simulink model "NewModel"  (R2018a)
settings: Solver=VariableStepAuto  StartTime=0.0  StopTime=10  RelTol=1e-3
values from neighbouring files (symbols this model uses):
  a22 = -2*beta*(c+f10)/numitor    (= -0.0723201373103)    [Proiect_script_IRA2.m]    (also in decupalre.m; trying.m)
  a23 = -M*g*L*f10/numitor    (= -43.7694067093)    [Proiect_script_IRA2.m]    (also in decupalre.m; trying.m)
  a24 = 2*beta*(c+f10)/numitor    (= 0.0723201373103)    [Proiect_script_IRA2.m]    (also in decupalre.m; trying.m)
  a42 = 2*beta*(d+f10)/numitor    (= 0.0279773616358)    [Proiect_script_IRA2.m]    (also in decupalre.m; trying.m)
  a43 = d*M*g*L/numitor    (= 43.7747367103)    [Proiect_script_IRA2.m]    (also in decupalre.m; trying.m)
  a44 = 2*beta*(d+f10)/numitor    (= 0.0279773616358)    [Proiect_script_IRA2.m]    (also in decupalre.m = -0.0279773616358; trying.m = -0.0279773616358)
  a66 = ((-W*W*beta)/(2*R*R))/(m*W*W/2+W*W/(2*R*R)*(Jw+Jm)+Jphi)    (= -0.112438053457)    [Proiect_script_IRA2.m]    (also in decupalre.m; trying.m)
  b21 = alfa*(c+f10)/numitor    (= 1.04508868945)    [Proiect_script_IRA2.m]    (also in decupalre.m; trying.m)
  b22 = alfa*(c+f10)/numitor    (= 1.04508868945)    [Proiect_script_IRA2.m]    (also in decupalre.m; trying.m)
  b41 = -alfa*(d+f10)/numitor    (= -0.404297133465)    [Proiect_script_IRA2.m]    (also in decupalre.m; trying.m)
  b42 = -alfa*(d+f10)/numitor    (= -0.404297133465)    [Proiect_script_IRA2.m]    (also in decupalre.m; trying.m)
  b61 = ((-W*alfa)/(2*R))/(m*W*W/2+W*W/(2*R*R)*(Jw+Jm)+Jphi)    (= -0.609310260785)    [Proiect_script_IRA2.m]    (also in decupalre.m; trying.m)
  b62 = ((-W*alfa)/(2*R))/(m*W*W/2+W*W/(2*R*R)*(Jw+Jm)+Jphi)    (= -0.609310260785)    [Proiect_script_IRA2.m]    (also in decupalre.m; trying.m)
settings Model: Creator=Andrei  LastModifiedBy=Andrei

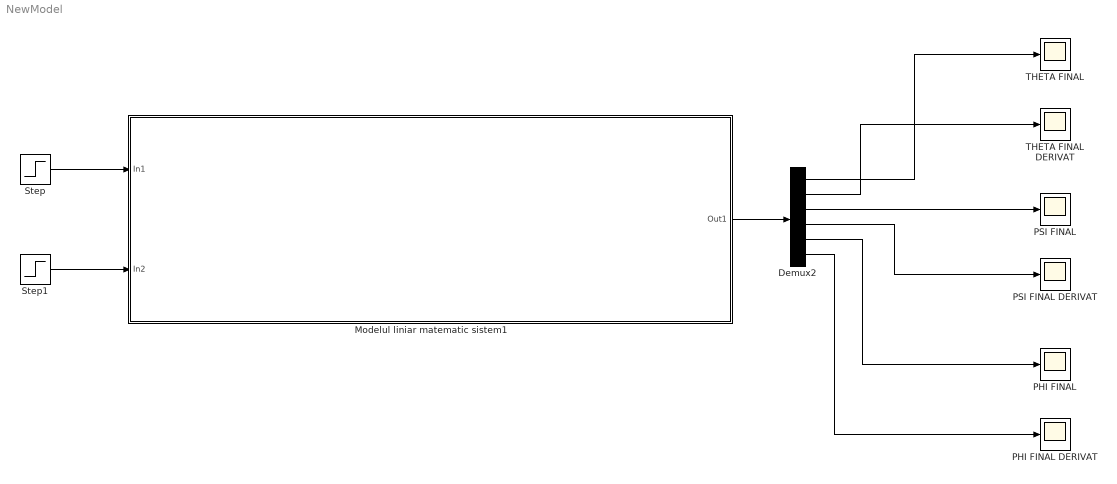
== system NewModel ==
  Demux2 : Demux  Outputs=6
  Modelul liniar matematic sistem1 : Subsystem
  PHI FINAL : Scope
  "PHI FINAL DERIVAT " : Scope
  PSI FINAL : Scope
  "PSI FINAL DERIVAT " : Scope
  Step : Step  Time=0  SampleTime=0
  Step1 : Step  Time=0  SampleTime=0
  THETA FINAL : Scope
  "THETA FINAL DERIVAT " : Scope
  wires:
  Demux2/1 -> THETA FINAL/1
  Demux2/2 -> "THETA FINAL DERIVAT "/1
  Demux2/3 -> PSI FINAL/1
  Modelul liniar matematic sistem1/1(Out1) -> Demux2/1
  Demux2/4 -> "PSI FINAL DERIVAT "/1
  Demux2/6 -> "PHI FINAL DERIVAT "/1
  Demux2/5 -> PHI FINAL/1
  Step/1 -> Modelul liniar matematic sistem1/1(In1)
  Step1/1 -> Modelul liniar matematic sistem1/2(In2)

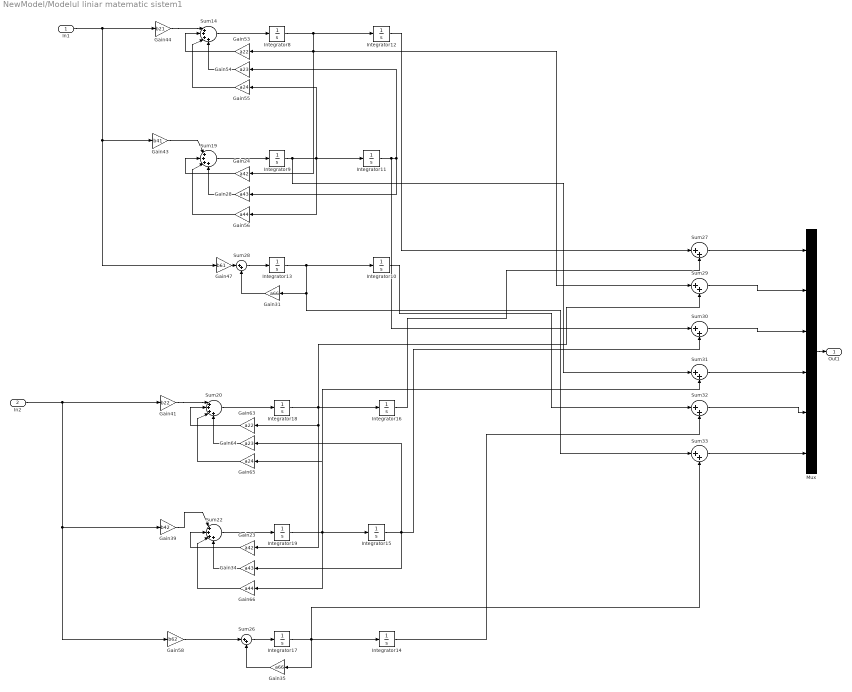
== system NewModel/Modelul liniar matematic sistem1 ==
  In1 : Inport
  In2 : Inport  Port=2
  Gain23 : Gain  Gain=a42
  Gain24 : Gain  Gain=a42
  Gain28 : Gain  Gain=a43
  Gain31 : Gain  Gain=a66
  Gain34 : Gain  Gain=a43
  Gain35 : Gain  Gain=a66
  Gain39 : Gain  Gain=b42
  Gain41 : Gain  Gain=b22
  Gain43 : Gain  Gain=b41
  Gain44 : Gain  Gain=b21
  Gain47 : Gain  Gain=b61
  Gain53 : Gain  Gain=a22
  Gain54 : Gain  Gain=a23
  Gain55 : Gain  Gain=a24
  Gain56 : Gain  Gain=a44
  Gain58 : Gain  Gain=b62
  Gain63 : Gain  Gain=a22
  Gain64 : Gain  Gain=a23
  Gain65 : Gain  Gain=a24
  Gain66 : Gain  Gain=a44
  Integrator{8..19} (12 alike) : Integrator
  Mux : Mux  Inputs=6
  Sum{14,19..20,22} (4 alike) : Sum  Inputs=|++++
  Sum{26..33} (8 alike) : Sum  Inputs=|++
  Out1 : Outport
  wires:
  Integrator9/1 -> Sum31/1, Gain56/1, Gain55/1, Integrator11/1
  Gain31/1 -> Sum28/2
  Gain66/1 -> Sum22/3
  Integrator19/1 -> Integrator15/1, Sum31/2, Gain66/1, Gain65/1
  Sum32/1 -> Mux/5
  Gain39/1 -> Sum22/1
  Gain55/1 -> Sum14/3
  Sum20/1 -> Integrator18/1
  Sum14/1 -> Integrator8/1
  Integrator17/1 -> Gain35/1, Integrator14/1, Sum33/2
  Sum30/1 -> Mux/3
  Gain44/1 -> Sum14/1
  Integrator8/1 -> Gain24/1, Sum29/1, Gain53/1, Integrator12/1
  Sum22/1 -> Integrator19/1
  Mux/1 -> Out1/1
  Integrator18/1 -> Sum29/2, Gain23/1, Gain63/1, Integrator16/1
  Gain24/1 -> Sum19/2
  Gain53/1 -> Sum14/2
  Sum19/1 -> Integrator9/1
  Sum33/1 -> Mux/6
  Gain64/1 -> Sum20/4
  Integrator14/1 -> Sum32/2
  Gain54/1 -> Sum14/4
  Integrator11/1 -> Sum30/1, Gain54/1, Gain28/1
  Integrator13/1 -> Sum33/1, Gain31/1, Integrator10/1
  Gain41/1 -> Sum20/1
  Gain34/1 -> Sum22/4
  Sum27/1 -> Mux/1
  Integrator16/1 -> Sum27/2
  Integrator15/1 -> Sum30/2, Gain64/1, Gain34/1
  Gain28/1 -> Sum19/4
  Gain47/1 -> Sum28/1
  Sum28/1 -> Integrator13/1
  Gain43/1 -> Sum19/1
  Gain35/1 -> Sum26/2
  Gain63/1 -> Sum20/2
  Gain23/1 -> Sum22/2
  Sum31/1 -> Mux/4
  Sum29/1 -> Mux/2
  Integrator12/1 -> Sum27/1
  Gain65/1 -> Sum20/3
  Gain56/1 -> Sum19/3
  Integrator10/1 -> Sum32/1
  Sum26/1 -> Integrator17/1
  Gain58/1 -> Sum26/1
  In1/1 -> Gain47/1, Gain43/1, Gain44/1
  In2/1 -> Gain39/1, Gain58/1, Gain41/1
